simulink library "Lib_Turbo_DuctQ_TMATS"  (Simulink 8.5)
settings: Solver=ode45  StartTime=0.0  StopTime=10.0  RelTol=1e-3
libraries: Lib_Thermo_Enth2Temp_TMATS x1, Lib_Thermo_Temp2Enth_TMATS x1
Description:
  | Thomas Modules
settings Model: Creator=jwchapm2  LastModifiedBy=jwchapm2

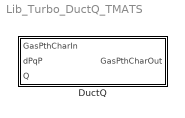
== system Lib_Turbo_DuctQ_TMATS ==
  DuctQ : Subsystem  mask(T-MATS: DuctQ Library Block){}
      mask help:
      | This block simulates the performance of a duct using basic fluid dynamic equations and properties.
      | With power and dPqP inputs.
      mask Help: web(which('Turbo_TMATS_DctQ.html'),'-helpbrowser')

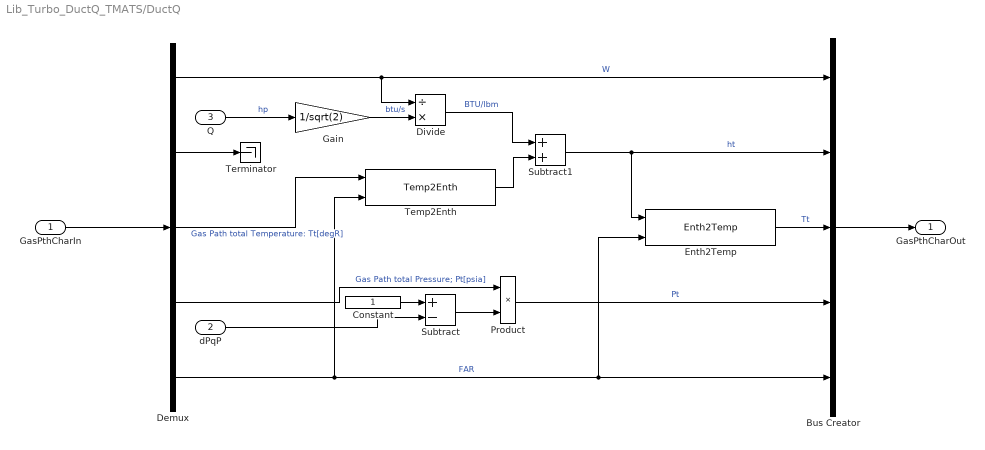
== system Lib_Turbo_DuctQ_TMATS/DuctQ ==
  GasPthCharIn : Inport
  dPqP : Inport  Port=2
  Q : Inport  Port=3
  Bus Creator : BusCreator  Inputs=5
  Constant : Constant
  Demux : Demux  Outputs=5
  Divide : Product  Inputs=/*
  Enth2Temp : Lib_Thermo_Enth2Temp_TMATS/Enth2Temp
  Gain : Gain  Gain=1/sqrt(2)
  Product : Product  RndMeth=Zero
  Subtract : Sum  Inputs=+-
  Subtract1 : Sum
  Temp2Enth : Lib_Thermo_Temp2Enth_TMATS/Temp2Enth
  Terminator : Terminator
  GasPthCharOut : Outport
  wires:
  Constant/1 -> Subtract/1
  dPqP/1 -> Subtract/2
  Demux/1 -> Divide/1, Bus Creator/1  "W"
  Demux/5 -> Temp2Enth/2, Enth2Temp/2, Bus Creator/5  "FAR"
  Demux/3 -> Temp2Enth/1  "Gas Path total Temperature: Tt[degR]"
  GasPthCharIn/1 -> Demux/1
  Bus Creator/1 -> GasPthCharOut/1
  Product/1 -> Bus Creator/4  "Pt"
  Demux/4 -> Product/1  "Gas Path total Pressure; Pt[psia]"
  Subtract/1 -> Product/2
  Subtract1/1 -> Bus Creator/2, Enth2Temp/1  "ht"
  Gain/1 -> Divide/2  "btu/s"
  Divide/1 -> Subtract1/1  "BTU/lbm"
  Q/1 -> Gain/1  "hp"
  Enth2Temp/1 -> Bus Creator/3  "Tt"
  Temp2Enth/1 -> Subtract1/2
  Demux/2 -> Terminator/1
